simulink model "Two_State_Model"  (R2019b)
settings: Solver=VariableStepAuto  StartTime=0.0  StopTime=10.0  RelTol=1e-3
settings Model: Creator=Lenovo  LastModifiedBy=Lenovo
settings OptimizationCC: DefaultParameterBehavior=Inlined

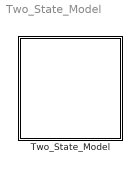
== system Two_State_Model ==
  Two_State_Model : Stateflow chart  BlockKeywords=__PRM__SERIALIZED__DATA__:Stateflow Chart,Stateflow Diagram  TreatAsAtomicUnit=on

== stateflow chart Two_State_Model/Two_State_Model ==
  state Entering_the_OTP
  state FINAL_PSEUDOSTATE
  state OTP_Validation
  state User_Authentication
  (default) -> Entering_the_OTP
  OTP_Validation -> Entering_the_OTP [order 1]
  User_Authentication -> FINAL_PSEUDOSTATE
  Entering_the_OTP -> OTP_Validation
  OTP_Validation -> User_Authentication [order 2]
